simulink library "powerlib2"  (Simulink 6.0)
settings: Solver=ode45  SolverMode=SingleTasking  StartTime=0.0  StopTime=10.0  RelTol=1e-3
undefined symbols (not defined in the file or in its folder): com, ctrl1, Da, DiscIntNeverNeededParam, dtha, etat, FA, gcbh, Ha, Ka, Lm, Ls, powericonV2, q0, Rm, Rs, sel, st_a, st_b, st_c, sta, stb, stc, T1, T2, T3, T4
libraries: powerlib2 x55, simulink_extras x5, powerlib_extras x4, powerlib_modelsV2 x4, simulink x1
(part 2 of 6)

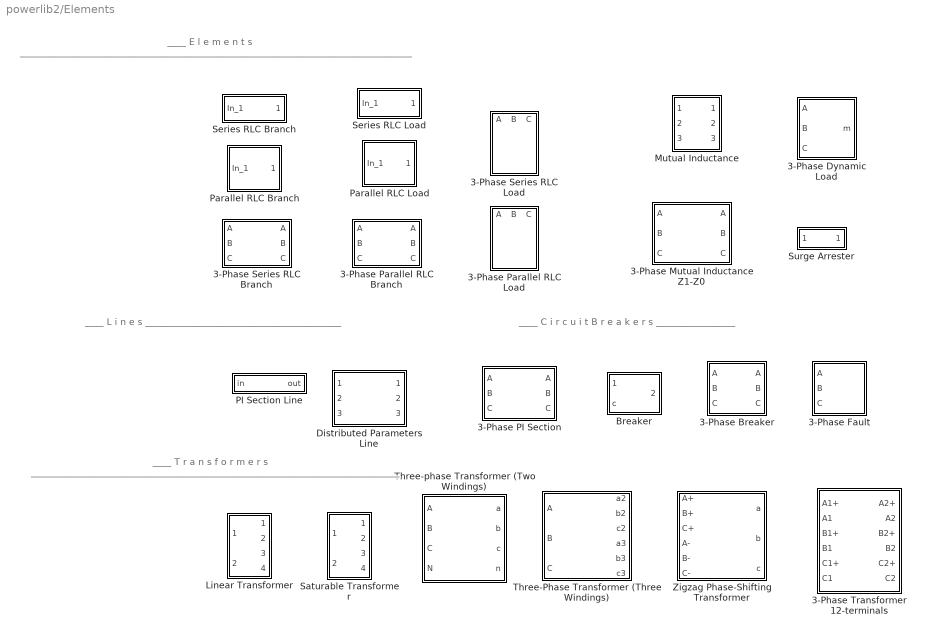
== system powerlib2/Elements ==
  note: ____ T r a n s f o r m e r s _______________________________________________________________________________
  note: ____ C i r c u i t B r e a k e r s _________________
  note: ____ E l e m e n t s ____________________________________________________________________________________
  note: ____ L i n e s __________________________________________
  3-Phase Dynamic Load : Subsystem  LoadFcn=powericonV2('psblfblk',bdroot,'gotofrom','Load');  mask(Three-Phase Dynamic Load){Vfnom=[ 500e3 60 ], PQ_0=[50e6 25e6], V0=[0.994 -11.8], PQext=off, n=[1.3 2], Tpq=[0  0  0  0], Vmin=0.7, LoadFlowParameters=[4,0,0,0,0]}
      mask prompts: Vfnom "Nominal L-L voltage and frequency  [Vn(Vrms) fn(Hz)]:"; PQ_0 "Active & reactive power at initial voltage [Po(W) Qo(var)]:"; V0 "Initial positive-sequence voltage Vo [Mag(pu) Phase (deg.)]:"; PQext "External control of PQ"; n "Parameters [ np  nq ]:"; Tpq "Time constants [Tp1 Tp2 Tq1 Tq2]  (s):"; Vmin "Minimum voltage Vmin (pu):"; LoadFlowParameters "Load Flow parameters"
      mask help:
      | Implements a three-phase, three-wire dynamic load. Active  power P and reactive power Q absorbed by the load vary as function of positive-sequence voltage V according to following equations:
      |
      |   If V>Vmin, P and Q vary as follows:
      |        P=Po*(V/Vo)^np*(1+Tp1.s)/(1+Tp2.s)
      |        Q=Qo*(V/Vo)^nq*(1+Tq1.s)/(1+Tq2.s)
      |   if V<Vmin
      |      Same equations with np=nq=2 (constant impedance load)
      |
      | Check 'External control of PQ'  to control power from a vectorized signal  [P Q] connected to input  4.
      | The m output returns a vector of 3 signals [V(pu) P(W) Q (var)].
      mask init:
      | powericonV2('psbcbtransfo',gcb,'3-Phase Dynamic Load')
      settings: CopyFcn=powericonV2('psblfblk',bdroot,'gotofrom','Copy');
      mask Help: web(psbhelp)
      mask CallbackString: |||powericonV2('psbcbtransfo',gcb,'3-Phase Dynamic Load',[]);||||
      mask Display:
      | plot(-45,-45,45,45,[0,9,18,24,29,30,29,24,18,9,0,-9,-18,-24,-29,-30,-29,-24,-18,-9,0]*.9,[30,29,24,18,9,0,-9,-18,-24,-29,-30,-29,-24,-18,-9,0,9,18,24,29,30]*.9)
      | plot([0,0,10,0,-10,0]*1.1,[15,-5,-5,-15,-5,-5]*1.1)
  3-Phase Mutual Inductance Z1-Z0 : Subsystem  mask(3-phase RL  positive & zero-sequence impedance){RL1=[ 2  50e-3], RL0=[4  100e-3]}
      mask prompts: RL1 "Positive-sequence parameters : [R1 (Ohms) L1 (H)]"; RL0 "Zero-sequence parameters :     [R0 (Ohms) L0 (H)]"
      mask help: This block implements a three phase impedance with mutual coupling between phases. Self impedances and mutual impedances are set by entering positive and zero sequences parameters.
      mask init:
      | [s1,s2,s3,s4,lp1,lp2,ls1,ls2,lt1,lt2,Rs,Ls,Rm,Lm]=powericonV2('3-phase RL  positive & zero-sequence impedance',RL1,RL0);
      mask Display: plot(s1,s2,s3,s4,lp1,lp2,ls1,ls2,lt1,lt2);
  3-Phase Parallel RLC Branch : Subsystem  mask(3-phase parallel RLC element ){R=1, L=1e-3, C=1e-6}
      mask prompts: R "Resistance R (Ohms):"; L "Inductance L (H):"; C "Capacitance C (F):"
      mask help: This block implements a three-phase parallel RLC branch. It uses three parallel RLC branch blocks.
      mask init:
      | [p0,p1,p2,p3,p4,p5,p6,p7,p8,p9,p10,p11,p12,p13,p14,p15] =powericonV2('3-phase parallel RLC element',R,L,C);
      mask Help: Look under the mask of the 3-phase parallel RLC element block to see how it is built
      mask Display: plot(p0-20,p1,p2+20,p3,p4,p5,p6,p7,p8,p9,p10,p11,p12,p13,p14,p15)
  3-Phase Parallel RLC Load : Subsystem  Orientation=down  mask(3-phase parallel RLC load ){Vpp=500e3, fn=60, P3=50e6, QL3=25e6, QC3=200e6}
      mask prompts: Vpp "Nominal phase-phase voltage (Vrms):"; fn "Nominal frequency (Hz):"; P3 "Three-phase active power P (W):"; QL3 "Three-phase inductive reactive power Ql (var)"; QC3 "Three-phase capacitive reactive power Qc (var) :"
      mask help: This block implements a three-phase parallel RLC load connected in Y configureation, with the neutral connected to the ground. Each phase consist of one parallel RLC load block connected between the phase input and the ground.
      mask init:
      | [p0,p1,p2,p3,p4,p5,p6,p7,p8,p9,p10,p11,p12,p13,p14,p15,p16] = powericonV2('3-phase parallel RLC load',P3,QL3,QC3);
      mask Help: Look under the mask of the 3-phase parallel RLC load block to see how it is built.
      mask Display: plot(p0-30,p1,p2,p3,p4,p5,p6,p7,p8,p9,p10,p11,p12,p13,p14,p15,[200,200],[-35 35],[215 215],[-25 25],[230 230],[-15 15],[p16,200],[0,0])
  "3-Phase Series RLC Branch " : Subsystem  mask(3-phase RLC series element){R=1, L=1e-3, C=1e-6}
      mask prompts: R "Resistance R (Ohms):"; L "Inductance L (H):"; C "Capacitance C (F):"
      mask help: This block implements a three-phase series RLC branch. It uses three series RLC branch blocks.
      mask init:
      | [p0,p1,p2,p3,p4,p5,p6,p7,p8,p9,p10,p11]=powericon('3-phase RLC series element',R,L,C);
      mask Help: Look under the mask of the 3-phase RLC series element block to see how it is built.
      mask Display: plot(p0-60,p1,p2+60,p3,p4,p5,p6,p7,p8,p9,p10,p11);
  3-Phase Series RLC Load : Subsystem  Orientation=down  mask(3-phase series RLC load ){Vpp=500e3, fn=60, P3=50e6, QL3=25e6, QC3=200e6}
      mask prompts: Vpp "Nominal phase-phase voltage (Vrms):"; fn "Nominal frequency (Hz):"; P3 "Three-phase active power P (W):"; QL3 "Three-phase inductive reactive power Ql (var)"; QC3 "Three-phase capacitive reactive power Qc (var) :"
      mask help: This block implements a three-phase series RLC load connected in Y configuration, with the neutral connected to the ground. Each phase consist of one series RLC load connected between the phase input and the ground.
      mask init:
      | [s1,s2,s3,s4,s5,s6,s7,s8,s9,s10,s11,s12,s13,s14,s15] = powericonV2('3-phase series RLC load',P3,QL3,QC3);
      mask Help: Look under the mask of the 3-phase series RLC load block to see how it is built
      mask Display: plot(s1-70,s2,s3,s4,s5,s6,s7,s8,s9,s10,s11,s12,s13,[-12,12],s14,[-7,7],s15,[-2,2]);
  3-Phase Breaker : Subsystem  mask(Three-Phase Breaker){init_states=open, sa=on, sb=on, sc=on, sw_times=[4/60  10/60], Ts=0, comext=off, Ron=0.001, Rp=1e6, Cp=inf, mesure=None}
      mask prompts: init_states "Initial status of breakers"; sa "Switching of phase A"; sb "Switching of Phase B"; sc "Switching of phase C"; sw_times "Transition times (s)"; Ts "Sample time of the internal timer Ts(s):"; comext "External control of switching times"; Ron "Breakers resistance Ron (ohms)"; Rp "Snubbers resistance Rp (Ohms)"; Cp "Snubbers capacitance Cp (Farad)"; mesure "Measurements"
      mask help: Connect this block in series with the three-phase element you want to switch. You can define the breaker timing directly from the dialog box or apply an external logical signal. If you check the 'External control' box, the external control input will appear.
      mask init:
      | [sta,stb,stc,etat,sw_times,switchings]=powericon('Three-Phase Breaker',init_states,sa,sb,sc,Ron,sw_times,comext);
      | if strcmp(init_states,'open')
      |     p3=75;
      | else
      |     p3=50;
      | end
      | p0=-10;
      | p1=110;
      | 
      | if Rp==inf | Cp==0 | (Rp==inf & Cp==0)
      |     s1 = 0;
      |     s2=0;
      | else
      |     s1=[20,20,40,40,60,60,80,80,80,60,60,40,40];
      |     s2=[45,30,30,35,35,30,30,45,30,30,25,25,30];
      | end
      | powericonV2('psbcbtransfo',gcb,'Three-phase Breaker');
      mask Help: web(psbhelp)
      mask StyleString: popup(open|closed),checkbox,checkbox,checkbox,edit,edit,checkbox,edit,edit,edit,popup(None|Breaker voltages|Breaker currents|Breaker voltages and currents)
      mask CallbackString: ||||||powericonV2('psbcbtransfo',gcb,'Three-phase Breaker')||||
      mask Display: plot(p0,0,p1,100,[15,15,25,25,15],[55,45,45,55,55],[75,75,85,85,75],[55,45,45,55,55],[25,75],[50,p3],s1,s2)
  3-Phase Fault : Subsystem  mask(Three-Phase Fault){sa=on, sb=on, sc=on, Rdef=0.001, st=on, Rt=0.001, comext=off, sw_status=[1 0], sw_times=[ 1/60 5/60], Ts=0, init_statext=[0 0 1], Rp=1e6, Cp=inf, mesure=None}
      mask prompts: sa "Phase A Fault"; sb "Phase B Fault"; sc "Phase C Fault"; Rdef "Fault resistances  Ron (ohms) :"; st "Ground Fault"; Rt "Ground resistance Rg (ohms) :"; comext "External control of fault timing :"; sw_status "Transition status [1,0,1 ...):"; sw_times "Transition times (s):"; Ts "Sample time of the internal timer Ts(s):"; init_statext "Initial status of fault [Phase A  Phase B  Phase C]:"; Rp "Snubbers resistance Rp (ohms) :"; Cp "Snubbers Capacitance Cp (Farad)"; mesure "Measurements"
      mask help: Use this block to program a fault (short-circuit) between any phase and the ground. You can define the fault timing directly from the dialog box or apply an external logical signal. If you check the 'External control' box , the external control input will appear.
      mask init:
      | [st_a,st_b,st_c,Rground,init_a,init_b,init_c,p7,p8,p9,p10,p11]=powericonV2('Three-Phase Fault',Rdef,Rt,sw_times,sw_status,sa,sb,sc,st,init_statext,comext);
      | desc0=setstr(p7);
      | desc1=setstr(p8);
      | desc2=setstr(p9);
      | desc3=setstr(p10);
      | desc4=setstr(p11);
      | powericonV2('psbcbtransfo',gcb,'Three-phase Fault');
      mask Help: web(psbhelp)
      mask StyleString: checkbox,checkbox,checkbox,edit,checkbox,edit,checkbox,edit,edit,edit,edit,edit,edit,popup(None|Fault voltages|Fault currents|Fault voltages and currents)
      mask CallbackString: ||||powericonV2('psbcbtransfo',gcb,'Three-phase Fault')||powericonV2('psbcbtransfo',gcb,'Three-phase Fault')|||||||
      mask Display: disp([desc0,'\n',desc1,desc2,desc3])
  3-Phase PI Section : Subsystem  mask(Three-phase transmission line pi-section){f=60, R10=[ 0.01273 0.3864], L10=[ 0.9337e-3  4.1264e-3], C10=[12.74e-9 7.751e-9], long=100}
      mask prompts: f "Frequency used for R L C specification (Hz) :"; R10 "Positive- and zero-sequence resistances  [R1 (Ohms/km)  R0 (Ohms/km) ] :"; L10 "Positive- and zero-sequence inductances [ L1(H/km)  L0 (H/km)] :"; C10 "Positive- and zero-sequence capacitances [ C1(F/km) C0(F/km)] :"; long "Line section length (km) :"
      mask help: This block implements a three-phase PI section line to represent a three-phase transmision line. This block represents only one PI section. To implements more that one PI section, you simply need to connect copies of this block in series.
      mask init:
      | [Rs,Ls,Rm,Lm,Cp,Cn] = powericonV2('Three-phase transmission line pi-section',f,R10,L10,C10,long);
      mask Help: Look under the mask of the Three-phase transmission line pi-section block to see how it is built.
      mask Display: plot(0,0,100,100,[20,20,80,80,90,80,80,20,20,10],[50,40,40,50,50,50,61,61,50,50],[56,39],[55,55],[44,44],[44,55],[53,50,50],[44,48,55])
  3-Phase Transformer 12-terminals : Subsystem  mask(Three-phase Linear Transformer 12-terminals){pf=[ 10e6 60 ], urx1=[ 10e3 0.002  0.05 ], urx2=[ 25e3 0.002 0.05], rxm=[ 200 200 ]}
      mask prompts: pf "[Three-phase rated power(VA)  Frequency (Hz)]"; urx1 "Winding 1 : [phase voltage(Vrms)  R(pu)  X(pu)] :"; urx2 "Winding 2 : [phase voltage(Vrms)  R(pu)  X(pu)] :"; rxm "Magnetizing branch : [Rm(pu)  Xm(pu)] :"
      mask help: This block implements three single-phase two-winding transformers . All winding terminals are accessible.
      mask init:
      | [p1,p2,p3,p4,p5,p6,p7,p8,p9,p10,p11,p12,p13,p14,p15,p16,p17,p18,p19,p20,p21,p22,p23,p24] = powericonV2('Three-phase Linear Transformer 12-terminals',pf,urx1,urx2);
      | pnom=pf(1)/3;
      |  fnom=pf(2);
      | u1=urx1(1);
      | r1=urx1(2);
      |  x1=urx1(3);
      | u2=urx2(1);
      | r2=urx2(2);
      |  x2=urx2(3);
      mask Help: Look under the mask of the Three-phase Linear Transformer 12-terminals block to see how it is built.
      mask Display: plot(-130,-100,130,100,p1,p2,p3,p4,p13,p14,p15,p16,      p5,p6,p7,p8, p17,p18,p19,p20,     p9,p10,p11,p12,p21,p22,p23,p24  )
  Breaker : Subsystem  Tag=PoWeRsYsTeMbLoCk  LoadFcn=powericonV2('psblfblk',bdroot,'goto','Load');  mask(Breaker){a=0.01, c=0, rs=1e6, cs=inf, times=[ 4/60  5/60 ], Ts=0, comext=on, mesure=None, PSBOutputType=1}
      mask prompts: a "Breaker resistance Ron (Ohm):"; c "Initial state ( 0 for 'open' , 1 for 'closed' ):"; rs "Snubber resistance Rs (Ohms):"; cs "Snubber capacitance Cs (F):"; times "Switching times (s):"; Ts "Sample time of the internal timer Ts(s):"; comext "External control of switching times"; mesure "Measurements"; PSBOutputType "Output type [1=PSB  0=simulink output]"
      mask help:
      | Implements a circuit breaker with internal resistance Ron (Ron, required by model , cannot be set to zero).
      | First input (1) and output (2) are the two  breaker terminals. 2nd input (c) is a Simulink logical signal controlling the breaker.  When  2nd input  becomes greater than zero the breaker closes instantaneously.  When 2nd input becomes zero, the breaker opens at the next current zero-crossing.
      mask init:
      | [p0,p1,p3,s1,s2,com,switchings]=powericonV2('Breaker',c,rs,cs,times,comext);
      | powericonV2('psbcbtransfo',gcb,'Single-phase Breaker');
      settings: CopyFcn=powericonV2('psblfblk',bdroot,'goto','Copy');
      mask Help: web(psbhelp);
      mask StyleString: edit,edit,edit,edit,edit,edit,checkbox,popup(None|Branch voltage|Branch current|Branch voltage and current),edit
      mask CallbackString: ||||||powericonV2('psbcbtransfo',gcb,'Single-phase Breaker')||
      mask Display: plot(p0,25,p1,75,[15,15,25,25,15],[55,45,45,55,55],[75,75,85,85,75],[55,45,45,55,55],[25,75],[50,p3],s1,s2)
  Distributed Parameters Line : Subsystem  Tag=PoWeRsYsTeMbLoCk  mask(Distributed Parameters Line){n=3, f=60, r=[0.01273 0.3864], l=[0.9337e-3  4.1264e-3], c=[12.74e-9 7.751e-9], lgt=300, x1=[0 0 0 0; 0.0001244 0 0 0; 0.0002488 0 0 0; 0.0003733 0 0 0; 0.0004977 0 0 0; 0.0006221 0 0 0], x2=[0 0 0 0; 0.0001244 0 0 0; 0.0002488 0 0 0; 0.0003733 0 0 0; 0.0004977 0 0 0; 0.0006221 0 0 0], x3=[0 0 0 0; 0.0001244 0 0 0; 0.0002488 0 0 0; 0.0003733 0 0 0; 0.0004977 0 0 0; 0.0006221 0 0 0], x4=[0 0 0 0; 0.0001244 0 0 0; 0.0002488 0 0 0; 0.0003733 0 0 0; 0.0004977 0 0 0; 0.0006221 0 0 0], x5=0, mesure=None, PSBOutputType=111111111111111111111111111111}
      mask prompts: n "Number of phases N"; f "Frequency used for R L C specification (Hz)"; r "Resistance per unit length (Ohms/km)   [N*N matrix] or [R1 R0 R0m]"; l "Inductance per unit length (H/km) [N*N matrix ] or [L1 L0 L0m]"; c "Capacitance per unit length (F/km) [N*N matrix] or [C1 C0 C0m]"; lgt "Line length (km)"; x1 "v1 init"; x2 "v2 init"; x3 "I1 init"; x4 "I2 init"; x5 "time delay init"; mesure "Measurements"; PSBOutputType "Output type [1=PSB  0=simulink output]"
      mask help:
      | Implements a N-phases distributed parameter line model. The R,L, and C line parameters are specified by [NxN] matrices.
      |
      | To model a two-, three-, or a six-phase symetrical line you can either specify complete [NxN] matrices or simply enter sequence parameters vectors: the  positive and zero sequence parameters for a two-phase or  three-phase transposed  line, plus the mutual zero-sequence for a  six-phase transposed  line  (2 coupled 3-phase lines).
      mask init:
      | [a1,a2,a3,a4,a5,a6,gx,gy]=powericonV2('Distributed Parameters Line',n);
      mask Help: web(psbhelp);
      mask StyleString: edit,edit,edit,edit,edit,edit,edit,edit,edit,edit,edit,popup(None|Phase-to-ground voltages),edit
      mask Display: plot(a1,a2,a3,a4,a5,a6,gx,gy,-10,0,110,120)
  Linear Transformer : Subsystem  Tag=PoWeRsYsTeMbLoCk  mask(Linear Transformer){a=[250e6 60], b=[735e3/sqrt(3) 0.002 0.08], c=[315e3/sqrt(3) 0.002 0.08], w3check=on, d=[60e3 0.005 0.02], e=[500 500], mesure=None, PSBOutputType=1111}
      mask prompts: a "Nominal power and frequency [Pn(VA) fn(Hz)]:"; b "Winding 1 parameters [V1(Vrms) R1(pu) L1(pu)]:"; c "Winding 2 parameters [V2(Vrms) R2(pu) L2(pu)]:"; w3check "Three windings transformer"; d "Winding 3 parameters [V3(Vrms) R3(pu) L3(pu)]:"; e "Magnetization resistance and reactance [Rm(pu) Lm(pu)]:"; mesure "Measurements"; PSBOutputType "Output type [1=PSB  0=simulink output]"
      mask help: Three windings linear transformer.
      mask init:
      | powericonV2('psbcbtransfo',gcb,'Linear Transformer'); [s1,s2,s3,s4,lpx,lpy,ls1x,ls1y,ls2x,ls2y,b1,b2,b3,b4] = powericonV2('Linear Transformer',w3check);
      settings: CopyFcn=powericonV2('psblfblk',bdroot,' ','Copy');
      mask Help: web(psbhelp);
      mask StyleString: edit,edit,edit,checkbox,edit,edit,popup(None|Winding voltages|Winding currents|Magnetization current|All voltages and currents),edit
      mask CallbackString: |||powericonV2('psbcbtransfo',gcb,'Linear Transformer');||||
      mask Display: plot(s1,s2,s3,s4,lpx,lpy,ls1x,ls1y,ls2x,ls2y,b1,b2,b3,b4)
  Mutual Inductance : Subsystem  Tag=PoWeRsYsTeMbLoCk  mask(Mutual Inductance){a=[1.1 1.1e-03], b=[ 1.1 1.1e-03], w3check=on, c=[ 1.1 1.1e-03], d=[1.0 1.0e-03], mesure=None, PSBOutputType=111}
      mask prompts: a "Winding 1 self impedance [R1(Ohm) L1(H)]:"; b "Winding 2 self impedance [R2(Ohm) L2(H)]:"; w3check "Three windings Mutual Inductance"; c "Winding 3 self impedance [R3(Ohm) L3(H)]:"; d "Mutual impedance [Rm(Ohm) Lm(H)]:"; mesure "Measurements"; PSBOutputType "Output type [1=PSB  0=simulink output]"
      mask help: Implements three inductances with mutual coupling.
      mask init:
      | powericonV2('psbcbtransfo',gcb,'Mutual Inductance'); [s1,s2,s3,s4,lp1,lp2,ls1,ls2,lt1,lt2,b1,b2,b3,b4] = powericonV2('Mutual Inductance',w3check);
      settings: CopyFcn=powericonV2('psblfblk',bdroot,' ','Copy');
      mask Help: web(psbhelp);
      mask StyleString: edit,edit,checkbox,edit,edit,popup(None|Winding voltages|Winding currents|Winding voltages and currents),edit
      mask CallbackString: ||powericonV2('psbcbtransfo',gcb,'Mutual Inductance');||||
      mask Display: plot(s1,s2,s3,s4,lp1,lp2,ls1,ls2,lt1,lt2,b1,b2,b3,b4)
  PI Section Line : Subsystem  Tag=PoWeRsYsTeMbLoCk  mask(Pi Section Line){f=60, a=0.2568, b=2e-03, c=8.6e-09, d=100, e=1, mesure=None, PSBOutputType=1}
      mask prompts: f "Frequency used for R L C specification (Hz)"; a "Resistance per unit length (Ohms/km):"; b "Inductance per unit length (H/km):"; c "Capacitance per unit length (F/km):"; d "Length (km):"; e "Number of pi sections:"; mesure "Measurements"; PSBOutputType "Output type [1=PSB  0=simulink output]"
      mask help: PI section transmission line.
      settings: CopyFcn=powericonV2('psblfblk',bdroot,' ','Copy');
      mask Help: web(psbhelp);
      mask StyleString: edit,edit,edit,edit,edit,edit,popup(None|Input and output voltages|Input and output currents|All voltages and currents),edit
      mask Display: plot(0,0,100,100,[45,45],[21,60],[54,41],[60,60],[50,49,49,49,49],[21,29,38,47,60])
  Parallel RLC Branch : Subsystem  Tag=PoWeRsYsTeMbLoCk  mask(Parallel RLC Branch){a=1, b=1e-03, c=1e-06, mesure=None, PSBOutputType=1}
      mask prompts: a "Resistance R (Ohms):"; b "Inductance L (H):"; c "Capacitance C (F):"; mesure "Measurements"; PSBOutputType "Output type [1=PSB  0=simulink output]"
      mask help: Implements a parallel RLC branch.
      mask init:
      | [s1,s2,s3,s4,r1,r2,l1,l2,c1,c2,c3,c4,x1,x2,x3,x4] = powericonV2('Parallel RLC Branch',a,b,c);
      settings: CopyFcn=powericonV2('psblfblk',bdroot,' ','Copy');
      mask Help: web(psbhelp);
      mask StyleString: edit,edit,edit,popup(None|Branch voltage|Branch current|Branch voltage and current),edit
      mask Display: plot(s1,s2,s3,s4,r1,r2,l1,l2,c1,c2,c3,c4,x1,x2,x3,x4)
  Parallel RLC Load : Subsystem  Tag=PoWeRsYsTeMbLoCk  mask(Parallel RLC Load){a=1000, b=60, c=10e3, d=100, e=100, mesure=None, PSBOutputType=1}
      mask prompts: a "Nominal voltage Vn (Vrms):"; b "Nominal frequency fn (Hz):"; c "Active power P (W):"; d "Inductive reactive Power QL (positive var):"; e "Capacitive reactive power Qc (negative var):"; mesure "Measurements"; PSBOutputType "Output type [1=PSB  0=simulink output]"
      mask help: Implements a parallel RLC load.
      mask init:
      | [s1,s2,s3,s4,r1,r2,l1,l2,c1,c2,c3,c4,x1,x2,x3,x4] = powericonV2('Parallel RLC Load',c,d,e);
      settings: CopyFcn=powericonV2('psblfblk',bdroot,' ','Copy');
      mask Help: web(psbhelp);
      mask StyleString: edit,edit,edit,edit,edit,popup(None|Branch voltage|Branch current|Branch voltage and current),edit
      mask Display: plot(s1,s2,s3,s4,r1,r2,l1,l2,c1,c2,c3,c4,x1,x2,x3,x4)
  Saturable Transformer : Subsystem  Tag=PoWeRsYsTeMbLoCk  mask(Saturable Transformer){a=[250e6 60], b=[735e3/sqrt(3) 0.002 0.08], c=[315e3/sqrt(3) 0.002 0.08], w3check=on, d=[315e3/sqrt(3) 0.002 0.08], e=[ 0,0 ; 0.0024,1.2 ; 1.0,1.52 ], f=[500], H=off, matfile='hysteresis', Initialslope=+1, mesure=None, PSBOutputType=1111}
      mask prompts: a "Nominal power and frequency [Pn(VA) fn(Hz)]:"; b "Winding 1 parameters [V1(Vrms) R1(pu) L1(pu)]:"; c "Winding 2 parameters [V2(Vrms) R2(pu) L2(pu)]:"; w3check "Three windings transformer"; d "Winding 3 parameters [V3(Vrms) R3(pu) L3(pu)]:"; e "Saturation characteristic [i1(pu) phi1(pu); i2 phi2; ...]:"; f "Core loss resistance and initial flux [Rm(pu) phi0(pu)] or [Rm(pu)] only:"; H "Simulate hysteresis"; matfile "Hysteresis Data Mat file"; Initialslope "Initial slope of flux"; mesure "Measurements"; PSBOutputType "Output type [1=PSB  0=simulink output]"
      mask help: Three winding saturable transformer.
      mask init:
      | powericonV2('psbcbtransfo',gcb,'Hysteresis'); [s1,s2,s3,s4,lpx,lpy,ls1x,ls1y,ls2x,ls2y,cx,cy] = powericonV2('Saturable Transformer',w3check);
      mask Help: web(psbhelp);
      mask StyleString: edit,edit,edit,checkbox,edit,edit,edit,checkbox,edit,popup(+1|-1),popup(None|Winding voltages|Winding currents|Flux and excitation current ( Imag+ IRm )|Flux and magnetization current ( Imag )|All measurements (V I Flux)),edit
      mask CallbackString: |||powericonV2('psbcbtransfo',gcb,'Hysteresis')||||powericonV2('psbcbtransfo',gcb,'Hysteresis')||||
      mask Display: plot(s1,s2,s3,s4,lpx,lpy,ls1x,ls1y,ls2x,ls2y,cx,cy)
  Series RLC Branch : Subsystem  Tag=PoWeRsYsTeMbLoCk  mask(Series RLC Branch){a=1, b=1e-03, c=1e-06, mesure=None, PSBOutputType=1}
      mask prompts: a "Resistance R (Ohms):"; b "Inductance L (H):"; c "Capacitance C (F):"; mesure "Measurements"; PSBOutputType "Output type [1=PSB  0=simulink output]"
      mask help: Implements a series RLC branch.
      mask init:
      | [s1,s2,s3,s4,r1,r2,l1,l2,c1,c2,c3,c4] = powericon('Series RLC Branch',a,b,c);
      settings: CopyFcn=powericonV2('psblfblk',bdroot,' ','Copy');
      mask Help: web(psbhelp);
      mask StyleString: edit,edit,edit,popup(None|Branch voltage|Branch current|Branch voltage and current),edit
      mask Display: plot(s1,s2,s3,s4,r1,r2,l1,l2,c1,c2,c3,c4)
  Series RLC Load : Subsystem  Tag=PoWeRsYsTeMbLoCk  mask(Series RLC Load){a=1000, b=60, c=10e3, d=100, e=100, mesure=None, PSBOutputType=1}
      mask prompts: a "Nominal voltage Vn (Vrms):"; b "Nominal frequency fn (Hz):"; c "Active power P (W):"; d "Inductive reactive power QL (positive var):"; e "Capacitive reactive power Qc (negative var):"; mesure "Measurements"; PSBOutputType "Output type [1=PSB  0=simulink output]"
      mask help: Implements a series RLC load.
      mask init:
      | [s1,s2,s3,s4,r1,r2,l1,l2,c1,c2,c3,c4] = powericon('Series RLC Load',c,d,e);
      settings: CopyFcn=powericonV2('psblfblk',bdroot,' ','Copy');
      mask Help: web(psbhelp);
      mask StyleString: edit,edit,edit,edit,edit,popup(None|Branch voltage|Branch current|Branch voltage and current),edit
      mask Display: plot(s1,s2,s3,s4,r1,r2,l1,l2,c1,c2,c3,c4)
  Surge Arrester : Subsystem  Tag=PoWeRsYsTeMbLoCk  mask(Surge Arrester){x1=500e+03, x2=2, x3=500, x4=[.955 50], x5=[1.0 25], x6=[.9915 16.5], mesure=None, PSBOutputType=1}
      mask prompts: x1 "Protection voltage  Vref(V):"; x2 "Number of columns:"; x3 "Reference current per column Iref(A):"; x4 "Segment 1 characteristics [ k1 alpha1 ]:"; x5 "Segment 2 characteristics [ k2 alpha2 ]:"; x6 "Segment 3 characteristics [ k3 alpha3 ]:"; mesure "Measurements"; PSBOutputType "Output type [1=PSB  0=simulink output]"
      mask help: Implements a metal-oxide surge arrester.
      mask Help: web(psbhelp);
      mask StyleString: edit,edit,edit,edit,edit,edit,popup(None|Branch voltage|Branch current|Branch voltage and current),edit
      mask Display: plot(-100,-45,100,45,[-100 -35],[0 0],[100 35],[0 0],[-30 -30],[40 -40],[-20 -20],[40 -40],[-10 -10],[40 -40],[0 0],[40 -40],[10 10],[-40 40],[20 20],[-40 40],[30 30],[-40 40])
  Three-Phase Transformer (Three Windings) : Subsystem  Tag=PoWeRsYsTeMbLoCk  mask(Three-Phase Transformer (Three Windings)){confi=ABC as input terminals, nom=[ 250e6 , 60 ], ydw1=Y, w1=[ 735e3 , 0.002 , 0.08 ], ydw2=Y, w2=[ 315e3 , 0.002 , 0.08 ], ydw3=Delta (D1), w3=[ 315e3 , 0.002 , 0.08 ], ynsat=off, rmag=500, lm=500, sat=[ 0,0 ; 0.0024,1.2 ; 1.0,1.52 ], hyst=off, matfile='hysteresis', sif=off, ifl=[0.8 -0.8 0.7], initialslopes=[+1 +1 +1], mesure=None, PSBOutputType=1111111}
      mask prompts: confi "Port Configuration"; nom "Nominal power and frequency  [ Pn(VA) , fn(Hz) ]"; ydw1 "Winding 1 (ABC) connection:"; w1 "Winding parameters [ V1 Ph-Ph(Vrms) , R1(pu) , L1(pu) ]"; ydw2 "Winding 2 (abc-2) connection:"; w2 "Winding parameters [ V2 Ph-Ph(Vrms) , R2(pu) , L2(pu) ]"; ydw3 "Winding 3 (abc-3) connection:"; w3 "Winding parameters [ V3 Ph-Ph(Vrms) , R3(pu) , L3(pu) ]"; ynsat "Saturable core"; rmag "Magnetization resistance  Rm(pu):"; lm "Magnetization reactance Lm(pu)"; sat "Saturation characteristic (pu) [  i1 phi1;  i2 phi2 ; ...]"; hyst "Simulate hysteresis"; matfile "Hysteresis Data Mat file"; sif "Specify initial fluxes:"; ifl "[ phi0A phi0B phi0C] (pu)"; initialslopes "Initial slopes of fluxes"; mesure "Measurements"
      mask help: This block implements a three-phase transformer by using three single-phase transformers. Set the winding connection to 'Yn' when you want to access the neutral point of the Wye (for winding 1 and 3 only).
      mask init:
      | if confi==2
      | p=-1;ofst=35;
      | else
      | p=1;ofst=0;
      | end;
      | if ydw1==1|ydw1==2|ydw1==3
      | w1x = [0,0,-5,0,5]*2.5-110;
      | w1y=[0,5,10,5,10]*3.2+40;
      | end
      | if ydw1==3
      | g1x=[0,1,1,0,0,1]*15-p*90+ofst;
      | g1y=[ 0,0,2,2,1,1]*15+30;
      | else
      | g1x=[];
      | g1y=[];
      | end
      | if ydw1==4|ydw1==5
      | w1x = [ 0,10,5,0 ]*2.5-92;
      | w1y=[0,0,10,0]*3+40;
      | end
      | if ydw2==1|ydw2==2
      | w2x=[0,0,-5,0,5]*2.5+65;
      | w2y=[0,5,10,5,10]*3.2+140;
      | end
      | if ydw2==2
      | g2x=[0,1,1,0,0,1]*15+p*80+ofst;
      | g2y=[ 0,0,2,2,1,1]*15+120;
      | else
      | g2x=[];
      | g2y=[];
      | end
      | if ydw2==3|ydw2==4
      | w2x=[0,10,5,0]*2.5+62;
      | w2y=[0,0,10,0]*3+90;
      | end
      | 
      | if ydw3==1|ydw3==2|ydw3==3
      | w3x=[0,0,-5,0,5]*2.5+65;
      | w3y=[0,5,10,5,10]*3.2-170;
      | end
      | if ydw3==3
      | g3x=[0,1,1,0,0,1]*15+p*80+ofst;
      | g3y=[ 0,0,2,2,1,1]*15-190;
      | else
      | g3x=[];
      | g3y=[];
      | end
      | if ydw3==4|ydw3==5
      | w3x=[0,10,5,0]*2.5+68;
      | w3y=[0,0,10,0]*3-40;
      | end
      | if ynsat==1
      | satx=[-50,-10,10,50];
      | saty=[-160,-160,160,160];
      | else
      | satx=[];
      | saty=[];
      | end
      | powericonV2('psbcbtransfo',gcb,'port configuration')
      | powericonV2('psbcbtransfo',gcb,'ThreeWindingsAccessToNeutrals',1);
      | powericonV2('psbcbtransfo',gcb,'ThreeWindingsAccessToNeutrals',3);
      mask Help: web(psbhelp);
      mask StyleString: popup(ABC as input terminals|ABC as output terminals),edit,popup(Y|Yn|Yg|Delta (D1)|Delta (D11)),edit,popup(Y|Yg|Delta (D1)|Delta (D11)),edit,popup(Y|Yn|Yg|Delta (D1)|Delta (D11)),edit,checkbox,edit,edit,edit,checkbox,edit,checkbox,edit,popup([+1 +1 +1]|[+1 +1 -1]|[+1 -1 +1]|[+1 -1 -1]|[-1 +1 +1]|[-1 +1 -1]|[-1 -1 +1]|[-1 -1 -1]),popup(None|Winding voltages|Winding currents|Fluxes and excitation currents ( Imag + IRm )|Fluxes and magnetization currents ( Imag )|All measurements (V I Fluxes)),edit
      mask CallbackString: powericonV2('psbcbtransfo',gcb,'port configuration');||powericonV2('psbcbtransfo',gcb,'ThreeWindingsAccessToNeutrals',1);||||powericonV2('psbcbtransfo',gcb,'ThreeWindingsAccessToNeutrals',3);||powericonV2('psbcbtransfo',gcb,'saturation3');||||powericonV2('psbcbtransfo',gcb,'Hysteresis3');||powericonV2('psbcbtransfo',gcb,'InitialFluxes3');||||
      mask Display:
      | plot(-180,-220,180,220,[-100,-40]*p,[0,0],[100,40]*p,[65,65],[100,40]*p,[-68,-68],
      | [-54 -38 -25 -17 -15 -19 -29 -43 -55 -54 -38 -25 -17 -15 -19 -29 -43 -55 -54 -38 -25 -17 -15 -19 -29 -43 -55 -54 -38 -25 -17 -15 -19 -29 -43 -55]*p,[-98 -98 -92 -84 -74 -64 -56 -51 -50 -50 -48 -42 -34 -24 -14 -6 -1 0 0 3 8 17 27 36 44 49 50 50 53 58 67 77 86 94 99 99],[54 38 25 17 15 19 29 43 55 54 38 25 17 15 19 29 43 55]*p,[-117 -117 -111 -103 -93 -83 -75 -70 -69 -69 -67 -61 -53 -43 -33 -25 -20 -19],[54 38 25 17 15 19 29 43 55 54 38 25 17 15 19 29 43 55]*p, [13 16 21 30 40 49 57 62 63 63 66 71 80 90 99 107 112 112],w1x*p,w1y,g1x,g1y,w2x*p,w2y,g2x,g2y,w3x*p,w3y,g3x,g3y,satx,saty)
  Three-phase Transformer (Two Windings) : Subsystem  Tag=PoWeRsYsTeMbLoCk  mask(Three-Phase Transformer (Two Windings)){nominal=[ 250e6 , 60 ], type1=Yn, params1=[ 424.35e3 , 0.002 , 0.08 ], type2=Yn, params2=[ 315e3 , 0.002 , 0.08 ], ynsat=off, rmag=500, lm=500, sat=[ 0,0 ; 0.0024,1.2 ; 1.0,1.52 ], hyst=off, matfile='hysteresis', sif=off, phi0=[ 0.8 , -0.8 , 0.7 ], initialslopes=[+1 +1 +1], mesure=None, PSBOutputType=1111}
      mask prompts: nominal "Nominal power and frequency  [ Pn(VA) , fn(Hz) ]"; type1 "Winding 1 (ABC) connection :"; params1 "Winding parameters [ V1 Ph-Ph(Vrms) , R1(pu) , L1(pu) ]"; type2 "Winding 2 (abc) connection :"; params2 "Winding parameters [ V2 Ph-Ph(Vrms) , R2(pu) , L2(pu) ]"; ynsat "Saturable core"; rmag "Magnetization resistance  Rm (pu)"; lm "Magnetization reactance Lm (pu)"; sat "Saturation characteristic (pu) [ i1 ,  phi1 ;  i2 , phi2 ; ... ]"; hyst "Simulate hysteresis"; matfile "Hysteresis Data Mat  file"; sif "Specify initial fluxes"; phi0 "[ phi0A , phi0B , phi0C ] (pu):"; initialslopes "Initial slopes of fluxes"; mesure "Measurements"
      mask help: This block implements a three-phase transformer by using three single-phase transformers. Set the winding connection to 'Yn' when you want to access the neutral point of the Wye.
      mask init:
      | if type1==1|type1==2|type1==3
      | w1x = [0,0,-5,0,5]*2.5-85;
      | w1y=[0,5,10,5,10]*3.2-175;
      | end
      | if type1==3
      | g1x=[0,1,1,0,0,1]*15-70;
      | g1y=[ 0,0,2,2,1,1]*15-190;
      | else
      | g1x=[];
      | g1y=[];
      | end
      | if type1==4|type1==5
      | w1x = [ 0,10,5,0 ]*2.5-92;
      | w1y=[0,0,10,0]*3-175;
      | end
      | if type2==1|type2==2|type2==3
      | w2x=[0,0,-5,0,5]*2.5+80;
      | w2y=[0,5,10,5,10]*3.2-175;
      | end
      | if type2==3
      | g2x=[0,1,1,0,0,1]*15+95;
      | g2y=[ 0,0,2,2,1,1]*15-190;
      | else
      | g2x=[];
      | g2y=[];
      | end
      | if type2==4|type2==5
      | w2x=[0,10,5,0]*2.5+62;
      | w2y=[0,0,10,0]*3-175;
      | end
      | if ynsat==1
      | satx=[-30,-10,10,30];
      | saty=[-150,-150,150,150];
      | else
      | satx=[];
      | saty=[];
      | end
      | powericonV2('psbcbtransfo',gcb,'TwoWindingsAccessToNeutrals',1);
      | powericonV2('psbcbtransfo',gcb,'TwoWindingsAccessToNeutrals',2);
      mask Help: web(psbhelp);
      mask StyleString: edit,popup(Y|Yn|Yg|Delta (D1)|Delta (D11)),edit,popup(Y|Yn|Yg|Delta (D1)|Delta (D11)),edit,checkbox,edit,edit,edit,checkbox,edit,checkbox,edit,popup([+1 +1 +1]|[+1 +1 -1]|[+1 -1 +1]|[+1 -1 -1]|[-1 +1 +1]|[-1 +1 -1]|[-1 -1 +1]|[-1 -1 -1]),popup(None|Winding voltages|Winding currents|Fluxes and excitation currents ( Imag + IRm )|Fluxes and magnetization currents ( Imag )|All measurements (V I Fluxes)),edit
      mask CallbackString: |powericonV2('psbcbtransfo',gcb,'TwoWindingsAccessToNeutrals',1);||powericonV2('psbcbtransfo',gcb,'TwoWindingsAccessToNeutrals',2);||powericonV2('psbcbtransfo',gcb,'saturation2');||||powericonV2('psbcbtransfo',gcb,'Hysteresis2');||powericonV2('psbcbtransfo',gcb,'InitialFluxes2');||||
      mask Display:
      | plot(-180,-220,180,220,[-100,-40],[0,0],[100,40],[0,0],
      | [2 42 74 94 100 90 66 30 0 2 42 74 94 100 90 66 30 0 2 42 74 94 100 90 66 30 0 2 42 74 94 100 90 66 30 0]*.4-55,[-45 -45 -34 -17 3 22 38 48 50 50 55 66 83 103 122 138 148 150 150 155 166 183 203 222 238 248 250 250 255 266 283 303 322 338 348 348]*0.5-75,[2 42 74 94 100 90 66 30 0 2 42 74 94 100 90 66 30 0 2 42 74 94 100 90 66 30 0 2 42 74 94 100 90 66 30 0]*-.4+55,[-45 -45 -34 -17 3 22 38 48 50 50 55 66 83 103 122 138 148 150 150 155 166 183 203 222 238 248 250 250 255 266 283 303 322 338 348 348]*0.5-75,w1x,w1y,g1x,g1y,w2x,w2y,g2x,g2y,satx,saty)
  Zigzag Phase-Shifting Transformer : Subsystem  Tag=PoWeRsYsTeMbLoCk  mask(Zig-Zag Phase-Shifting Transformer){pfnom=[ 100e6 60], uprim=10e3, uphisec=[ 30e3  +15], conex=Yg, rx1=[ 0.0032 0.08 ], rx2=[ 0.002  0.08 ], rx3=[ 0.002 0.08 ], satcheck=off, rxm=[ 500 500 ], rmag=500, saturation=[ 0,0 ; 0.0024,1.2 ; 1.0,1.52 ], mesure=None, PSBOutputType=111}
      mask prompts: pfnom "Nominal power and frequency [Pn(VA)  fn (Hz)] :"; uprim "Primary (zig-zag) nominal voltage Vp (VrmsPh-Ph) :"; uphisec "Secondary nom. voltage & phase shift [V3(VrmsPh-Ph) Phi(Deg)]:"; conex "Secondary winding (abc) connection :"; rx1 "Winding 1 (zig-zag) : [ R1(pu)  L1(pu)] :"; rx2 "Winding 2 (zig-zag) : [ R2(pu)  L2(pu)] :"; rx3 "Winding 3 (secondary) :  [ R3(pu)  L3(pu)] :"; satcheck "Saturable core"; rxm "Magnetizing branch : [Rm(pu)  Lm(pu)] :"; rmag "Magnetization resistance  Rm (pu)"; saturation "Saturation characteristic (pu) [ i1 ,  phi1 ;  i2 , phi2 ; ... ]"; mesure "Measurements"
      mask help: This block implements a three-phase phase-shifting transformer by using three single-phase three-winding transformers. Primary consists of windings 1 and 2 connected in zig-zag. All primary terminals are accessible. Secondary (winding 3) can be connected in wye or delta.
      mask init:
      | alpha_deg=uphisec(2);
      | if  alpha_deg==0,
      |    errordlg(' Phase shift cannot be zero' , 'Parameter error');
      | end
      | if  abs(alpha_deg)>=120,
      |    errordlg(' Phase shift cannot be larger than or equal to 120 degrees' , 'Parameter error');
      | end
      | if alpha_deg>0
      |   % Drawing of winding 2 of Zig-Zag ; alpha>0
      |    pzx1= [34 42]; pzy1=[65 59];
      |    pzx2= [49 42]; pzy2=[37 30];
      |    pzx3= [19 19]; pzy3=[37 47];
      | else
      |    pzx1= [26 34]; pzy1=[59 65];
      |    pzx2= [49 49]; pzy2=[37 47];
      |    pzx3= [19 26]; pzy3=[37 30];
      | end
      | if conex(1)=='Y', % Wye connexion
      |   px1=[55,70,70]; py1=[37,50,65]; px2=[70,85];   py2=[50,37];
      | else % Delta connexion
      |   px1=[60,60,77,60]; py1=[65,35,50,65]; px2=[]; py2=[];
      | end
      | if strcmp(conex,'Yg')
      | % Ground drawing
      |   pgx1=[70,70]; pgy1=[50,40]; pgx2=[63,77]; pgy2=[40,40];
      |   pgx3=[65,75]; pgy3=[38,38]; pgx4=[67,73]; pgy4=[35,35];
      | else
      |   pgx1=[]; pgy1=[]; pgx2=[]; pgy2=[];
      |   pgx3=[]; pgy3=[]; pgx4=[]; pgy4=[];
      | end
      | powericonV2('psbcbtransfo',gcb,'ZigZagSecondaryWinding',0);
      mask Help: web(psbhelp)
      mask StyleString: edit,edit,edit,popup(Y|Yn|Yg|Delta D1(-30 deg.)|Delta D11(+30 deg.)),edit,edit,edit,checkbox,edit,edit,edit,popup(None|Phase voltages|Phase currents|Fluxes and excitation currents (Imag + IRm)|Fluxes and magnetization currents (Imag)|All measurements (V I Fluxes)),edit
      mask CallbackString: |||powericonV2('psbcbtransfo',gcb,'ZigZagSecondaryWinding',0);||||powericonV2('psbcbtransfo',gcb,'ZigZagSaturation',0);|||||
      mask Display:
      | plot(0,0,100,100,[19 31] ,[37 47], [49 37], [37 47], [34 34],[53 65]);
      | plot(0,0,100,100,pzx1,pzy1,pzx2,pzy2,pzx3,pzy3);
      | plot(0,0,100,100,px1,py1,px2,py2)                        plot(0,0,100,100,pgx1,pgy1,pgx2,pgy2,pgx3,pgy3,pgx4,pgy4)

== system powerlib2/Extra Library ==
